simulink model "sampleModel1836"  (R2023a)
settings: Solver=VariableStepAuto  StartTime=0.0  StopTime=10.0  RelTol=1e-3
libraries: hdlsllib x10, simulink x3
settings Model: Creator=user1  LastModifiedBy=user1

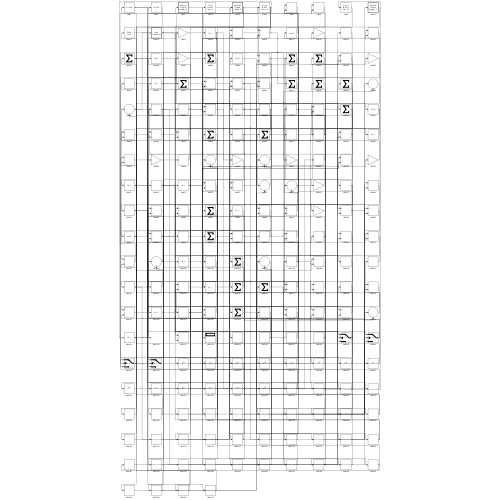
[thumbnail: Simulink's stored preview of the top-level diagram]
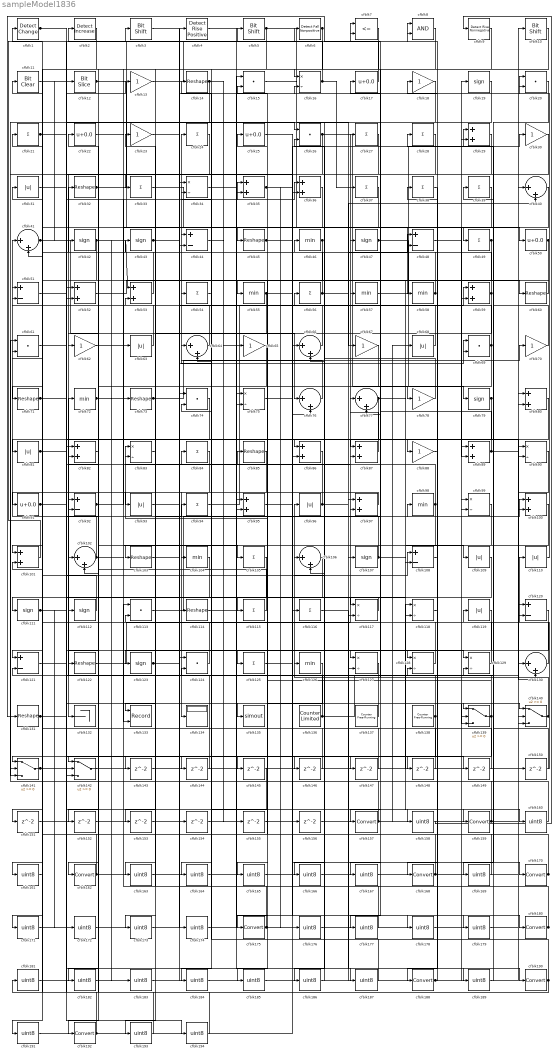
== system sampleModel1836 ==
  cfblk1 : simulink/Logic and Bit Operations/Detect Change  vinit=0  OutDataTypeStr=boolean
      settings: LibrarySourceBlock=|
      | hdlsllib/Logic and Bit
      | Operations/Detect
      | Change
  cfblk10 : hdlsllib/Logic and Bit Operations/Bit Shift  mode=Shift Left Logical  N=0
  cfblk{29,35..36,52..53,59,80,82,86..87,89,95,97,100..101} (15 alike) : Sum
  cfblk{40..41,64,66,76..77,102,106,130} (9 alike) : Sum  Inputs=|++
  cfblk{14,32,45,60,71,73,85,103,114,122,131} (11 alike) : Reshape
  cfblk{46,55,57..58,72,98,104,126} (8 alike) : MinMax
  cfblk{21,24,27..28,33,37..39,49,54,56,84,94,105,115..116,125} (17 alike) : Sum  Inputs=+
  cfblk{19,42..43,47,79,107,111..112,123} (9 alike) : Signum
  cfblk{44,48,51,92,108,120..121} (7 alike) : Sum  Inputs=+-
  cfblk{31,63,68,81,93,96,109..110,119} (9 alike) : Abs  SaturateOnIntegerOverflow=off
  cfblk11 : simulink/Logic and Bit Operations/Bit Clear  iBit=0
      settings: LibrarySourceBlock=|
      | hdlsllib/Logic and Bit
      | Operations/Bit Clear
  cfblk{15,20,26,61,69,74,113,124} (8 alike) : DotProduct  OutDataTypeStr=Inherit: Inherit via internal rule
  cfblk{16,34,75,83,90,99,117..118,127..129} (11 alike) : Product  Inputs=*/  RndMeth=Zero  SaturateOnIntegerOverflow=on
  cfblk12 : hdlsllib/Logic and Bit Operations/Bit Slice  lidx=7  ridx=0
  cfblk{13,18,23,30,62,65,67,70,78,88} (10 alike) : Gain
  cfblk132 : Terminator
  cfblk133 : Record  FileSettingsInternal="{\"entries\":[{\"content\":{\"excelSettings\":{\"content\":{},\"type\":\"Streamout.ExcelSettings\"}},\"type\":\"Streamout.FileSettingStorage\",\"uuid\":\"\"}],\"packageUris\":[\"http:\\/\\/schema.mathworks.com\\/mf0\\/streamout_blocks\\/R2020a\"],\"version\":\"1.0\"}"  Layout=[1 1]  SignalsInternal="{\"entries\":[{\"content\":{\"signals\":[{\"content\":{\"blockPath\":[],\"dimensions\":[1],\"domain\":\"\",\"lineColor\":\"#a2142f\",\"plots\":[1],\"port\":1,\"signalID\":4473,\"signalName\":\"XY Graph:1\"},\"type\":\"RecordBlkView.Signal\",\"uuid\":\"\"},{\"content\":{\"blockPath\":[],\"dimensions\":[1],\"domain\":\"\",\"lineColor\":\"#139fff\",\"plots\":[1],\"port\":2,\"signalID\":4476,\"signalName\":\"XY Graph:2\"},\"type\":\"RecordBlkView.Signal\",\"uuid\":\"\"}]},\"type\":\"RecordBlkView.InputSignals\",\"uuid\":\"\"}],\"packageUris\":[\"http:\\/\\/schema.mathworks.com\\/mf0\\/streamout_blocks\\/R2020a\"],\"version\":\"1.0\"}"  VisualizationBindings="{\"xyplotplugin\":{\"info\":[{\"series\":[{\"bindingParametersList\":[{\"parameter\":\"X-Axis\",\"signalID\":4473,\"signalName\":\"XY Graph:1\"},{\"parameter\":\"Y-Axis\",\"signalID\":4476,\"signalName\":\"XY Graph:2\"}],\"seriesID\":47126}],\"subplotID\":1}]}}"  CompatibilityTag=XY  st=-1
  cfblk134 : Display
  cfblk135 : ToWorkspace  VariableName=simout  SaveFormat=Timeseries  SampleTime=-1
  cfblk136 : hdlsllib/Sources/Counter Limited  uplimit=7  tsamp=-1
  cfblk137 : hdlsllib/Sources/Counter Free-Running  NumBits=16  tsamp=-1
  cfblk138 : hdlsllib/Sources/Counter Free-Running  NumBits=16  tsamp=-1
  cfblk{139..142} (4 alike) : Switch  SaturateOnIntegerOverflow=off  InputSameDT=off
  cfblk{143..156} (14 alike) : Delay  SampleTime=1
  cfblk{157,159,162,168,170,175,180,188,190,192} (10 alike) : DataTypeConversion  SaturateOnIntegerOverflow=off  RndMeth=Floor
  cfblk{158,160..161,163..167,169,171..174,176..179,181..187,189,191,193..194} (28 alike) : DataTypeConversion  OutDataTypeStr=uint8  SaturateOnIntegerOverflow=off  RndMeth=Floor
  cfblk{17,22,25,50,91} (5 alike) : Bias  Bias=0.0  SaturateOnIntegerOverflow=off
  cfblk2 : simulink/Logic and Bit Operations/Detect Increase  vinit=0.0  OutDataTypeStr=boolean
      settings: LibrarySourceBlock=|
      | hdlsllib/Logic and Bit
      | Operations/Detect
      | Increase
  cfblk3 : hdlsllib/Logic and Bit Operations/Bit Shift  mode=Shift Left Logical  N=0
  cfblk4 : hdlsllib/Logic and Bit Operations/Detect Rise Positive  vinit=0  OutDataTypeStr=boolean
  cfblk5 : hdlsllib/Logic and Bit Operations/Bit Shift  mode=Shift Left Logical  N=0
  cfblk6 : hdlsllib/Logic and Bit Operations/Detect Fall Nonpositive  vinit=0  OutDataTypeStr=boolean
  cfblk7 : RelationalOperator  Operator=<=  OutDataTypeStr=boolean  InputSameDT=off
  cfblk8 : Logic  AllPortsSameDT=off  OutDataTypeStr=boolean
  cfblk9 : hdlsllib/Logic and Bit Operations/Detect Rise Nonnegative  vinit=0  OutDataTypeStr=boolean
  wires:
  cfblk94/1 -> cfblk59/1
  cfblk140/1 -> cfblk96/1, cfblk17/1
  cfblk70/1 -> cfblk28/1
  cfblk72/1 -> cfblk139/3, cfblk140/1, cfblk183/1
  cfblk89/1 -> cfblk128/1, cfblk7/1, cfblk130/2
  cfblk102/1 -> cfblk41/1, cfblk135/1
  cfblk5/1 -> cfblk49/1, cfblk33/1, cfblk133/2
  cfblk28/1 -> cfblk132/1
  cfblk53/1 -> cfblk32/1
  cfblk101/1 -> cfblk3/1
  cfblk115/1 -> cfblk51/1
  cfblk76/1 -> cfblk24/1
  cfblk44/1 -> cfblk65/1
  cfblk23/1 -> cfblk50/1
  cfblk139/1 -> cfblk83/1, cfblk97/2, cfblk151/1
  cfblk52/1 -> cfblk60/1
  cfblk86/1 -> cfblk134/1
  cfblk97/1 -> cfblk93/1
  cfblk32/1 -> cfblk5/1, cfblk105/1
  cfblk124/1 -> cfblk72/1
  cfblk116/1 -> cfblk190/1
  cfblk92/1 -> cfblk35/1, cfblk127/1
  cfblk73/1 -> cfblk70/1, cfblk69/1
  cfblk113/1 -> cfblk100/1
  cfblk47/1 -> cfblk79/1, cfblk167/1
  cfblk17/1 -> cfblk131/1
  cfblk60/1 -> cfblk55/1
  cfblk131/1 -> cfblk94/1, cfblk128/2
  cfblk26/1 -> cfblk78/1, cfblk141/2
  cfblk4/1 -> cfblk180/1
  cfblk56/1 -> cfblk25/1, cfblk40/2
  cfblk96/1 -> cfblk91/1, cfblk48/1
  cfblk49/1 -> cfblk81/1, cfblk152/1
  cfblk57/1 -> cfblk29/1
  cfblk50/1 -> cfblk88/1, cfblk108/2
  cfblk7/1 -> cfblk62/1
  cfblk36/1 -> cfblk101/1
  cfblk78/1 -> cfblk46/1
  cfblk63/1 -> cfblk22/1
  cfblk41/1 -> cfblk76/1, cfblk12/1
  cfblk66/1 -> cfblk44/1
  cfblk54/1 -> cfblk114/1
  cfblk14/1 -> cfblk142/1, cfblk141/3, cfblk155/1
  cfblk13/1 -> cfblk6/1
  cfblk117/1 -> cfblk115/1
  cfblk87/1 -> cfblk27/1
  cfblk59/1 -> cfblk14/1, cfblk123/1
  cfblk91/1 -> cfblk111/1, cfblk87/2
  cfblk68/1 -> cfblk47/1
  cfblk16/1 -> cfblk2/1, cfblk37/1
  cfblk118/1 -> cfblk18/1
  cfblk114/1 -> cfblk98/1
  cfblk129/1 -> cfblk57/1
  cfblk98/1 -> cfblk83/2, cfblk153/1
  cfblk9/1 -> cfblk157/1
  cfblk2/1 -> cfblk121/1
  cfblk37/1 -> cfblk103/1
  cfblk137/1 -> cfblk102/1
  cfblk138/1 -> cfblk85/1, cfblk142/3
  cfblk142/1 -> cfblk110/1
  cfblk85/1 -> cfblk112/1
  cfblk42/1 -> cfblk53/1, cfblk73/1, cfblk71/1
  cfblk141/1 -> cfblk36/1, cfblk108/1
  cfblk136/1 -> cfblk10/1, cfblk92/2
  cfblk38/1 -> cfblk168/1
  cfblk48/1 -> cfblk89/1
  cfblk64/1 -> cfblk42/1
  cfblk1/1 -> cfblk26/1, cfblk127/2
  cfblk81/1 -> cfblk117/1, cfblk146/1
  cfblk69/1 -> cfblk54/1, cfblk104/1
  cfblk27/1 -> cfblk86/1
  cfblk58/1 -> cfblk31/1, cfblk7/2
  cfblk110/1 -> cfblk20/1
  cfblk21/1 -> cfblk139/1, cfblk36/2
  cfblk107/1 -> cfblk43/1, cfblk160/1
  cfblk62/1 -> cfblk63/1
  cfblk40/1 -> cfblk44/2
  cfblk123/1 -> cfblk56/1, cfblk69/2
  cfblk90/1 -> cfblk100/2
  cfblk10/1 -> cfblk52/2
  cfblk74/1 -> cfblk162/1
  cfblk12/1 -> cfblk58/1, cfblk45/1
  cfblk122/1 -> cfblk77/1
  cfblk39/1 -> cfblk188/1
  cfblk126/1 -> cfblk175/1
  cfblk93/1 -> cfblk20/2
  cfblk79/1 -> cfblk86/2, cfblk171/1
  cfblk82/1 -> cfblk192/1
  cfblk125/1 -> cfblk76/2
  cfblk71/1 -> cfblk90/2, cfblk8/2
  cfblk95/1 -> cfblk170/1
  cfblk33/1 -> cfblk89/2
  cfblk43/1 -> cfblk118/2, cfblk16/2
  cfblk65/1 -> cfblk122/1
  cfblk88/1 -> cfblk8/1
  cfblk61/1 -> cfblk159/1
  cfblk121/1 -> cfblk129/1
  cfblk30/1 -> cfblk77/2
  cfblk111/1 -> cfblk13/1, cfblk172/1
  cfblk15/1 -> cfblk67/1
  cfblk6/1 -> cfblk16/1, cfblk161/1, cfblk164/1
  cfblk130/1 -> cfblk21/1
  cfblk83/1 -> cfblk133/1
  cfblk127/1 -> cfblk121/2
  cfblk75/1 -> cfblk30/1
  cfblk46/1 -> cfblk102/2, cfblk125/1
  cfblk128/1 -> cfblk23/1
  cfblk35/1 -> cfblk176/1, cfblk178/1
  cfblk22/1 -> cfblk139/2
  cfblk77/1 -> cfblk109/1, cfblk144/1
  cfblk55/1 -> cfblk75/2, cfblk149/1
  cfblk18/1 -> cfblk66/2
  cfblk104/1 -> cfblk141/1
  cfblk45/1 -> cfblk87/1, cfblk179/1
  cfblk112/1 -> cfblk41/2
  cfblk24/1 -> cfblk92/1
  cfblk19/1 -> cfblk143/1
  cfblk143/1 -> cfblk118/1
  cfblk144/1 -> cfblk1/1
  cfblk100/1 -> cfblk145/1
  cfblk146/1 -> cfblk64/1
  cfblk8/1 -> cfblk147/1
  cfblk147/1 -> cfblk26/2
  cfblk108/1 -> cfblk148/1
  cfblk148/1 -> cfblk51/2
  cfblk149/1 -> cfblk97/1
  cfblk150/1 -> cfblk129/2
  cfblk151/1 -> cfblk117/2
  cfblk152/1 -> cfblk29/2
  cfblk153/1 -> cfblk124/1
  cfblk103/1 -> cfblk154/1
  cfblk154/1 -> cfblk35/2
  cfblk155/1 -> cfblk140/3
  cfblk25/1 -> cfblk156/1
  cfblk156/1 -> cfblk59/2
  cfblk157/1 -> cfblk34/1, cfblk142/2, cfblk68/1
  cfblk11/1 -> cfblk158/1
  cfblk158/1 -> cfblk9/1
  cfblk159/1 -> cfblk53/2, cfblk119/1
  cfblk160/1 -> cfblk61/1
  cfblk161/1 -> cfblk61/2
  cfblk162/1 -> cfblk130/1, cfblk11/1
  cfblk119/1 -> cfblk163/1
  cfblk163/1 -> cfblk74/1
  cfblk164/1 -> cfblk74/2
  cfblk120/1 -> cfblk165/1
  cfblk165/1 -> cfblk40/1
  cfblk67/1 -> cfblk166/1
  cfblk166/1 -> cfblk120/1
  cfblk167/1 -> cfblk120/2
  cfblk168/1 -> cfblk150/1, cfblk52/1
  cfblk20/1 -> cfblk169/1
  cfblk169/1 -> cfblk38/1
  cfblk170/1 -> cfblk75/1, cfblk15/2
  cfblk171/1 -> cfblk95/1
  cfblk172/1 -> cfblk95/2
  cfblk84/1 -> cfblk173/1
  cfblk173/1 -> cfblk15/1
  cfblk3/1 -> cfblk174/1
  cfblk174/1 -> cfblk84/1
  cfblk175/1 -> cfblk140/2, cfblk124/2
  cfblk176/1 -> cfblk126/1
  cfblk80/1 -> cfblk177/1
  cfblk177/1 -> cfblk113/2
  cfblk178/1 -> cfblk80/1
  cfblk179/1 -> cfblk80/2
  cfblk180/1 -> cfblk64/2, cfblk113/1
  cfblk181/1 -> cfblk4/1
  cfblk99/1 -> cfblk182/1
  cfblk182/1 -> cfblk107/1
  cfblk183/1 -> cfblk99/1
  cfblk145/1 -> cfblk184/1
  cfblk184/1 -> cfblk99/2
  cfblk106/1 -> cfblk185/1
  cfblk185/1 -> cfblk19/1
  cfblk109/1 -> cfblk186/1
  cfblk186/1 -> cfblk106/1
  cfblk34/1 -> cfblk187/1
  cfblk187/1 -> cfblk106/2
  cfblk188/1 -> cfblk48/2, cfblk90/1
  cfblk51/1 -> cfblk189/1
  cfblk189/1 -> cfblk39/1
  cfblk190/1 -> cfblk181/1, cfblk34/2
  cfblk29/1 -> cfblk191/1
  cfblk191/1 -> cfblk116/1
  cfblk192/1 -> cfblk101/2, cfblk66/1
  cfblk105/1 -> cfblk193/1
  cfblk193/1 -> cfblk82/1
  cfblk31/1 -> cfblk194/1
  cfblk194/1 -> cfblk82/2
